simulink model "codercheck"  (R2019b)
settings: Solver=VariableStepAuto  StartTime=0.0  StopTime=inf  RelTol=1e-3
settings Model: Creator=giull  LastModifiedBy=giull

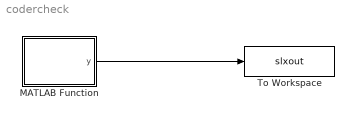
== system codercheck ==
  MATLAB Function : MATLAB Function  TreatAsAtomicUnit=on
  To Workspace : ToWorkspace  VariableName=slxout  SaveFormat=Timeseries  SampleTime=-1
  wires:
  MATLAB Function/1(y) -> To Workspace/1

== matlab function codercheck/MATLAB Function ==
  data: y output
function y  = MBfnc
persistent counter strArray
y=1;
if isempty(counter)
    counter = 1;
    
end

if isempty(strArray)
    strArray = [struct('a',multiObjectTracker,'b',multiObjectTracker)];
end

obj = multiObjectTracker();
cellOfObj = {obj; obj};

if isempty(cellOfObj)
    element = struct('a',multiObjectTracker,'b',multiObjectTracker);
elseif numel(cellOfObj)==1
    element = struct('a',cellOfObj{1,1},'b',multiObjectTracker);
elseif numel(cellOfObj)==2
    element = struct('a',cellOfObj{1,1},'b',multiObjectTracker);
end

strArrayOut = [strArray element];
%strArrayOut = strArray    
counter = counter + 1;   
end
